simulink model "Bai6"  (R2019a)
settings: Solver=VariableStepAuto  StartTime=0.0  StopTime=10  RelTol=1e-3
libraries: commanabbnd3 x1
settings Model: Creator=ASUS  LastModifiedBy=ASUS

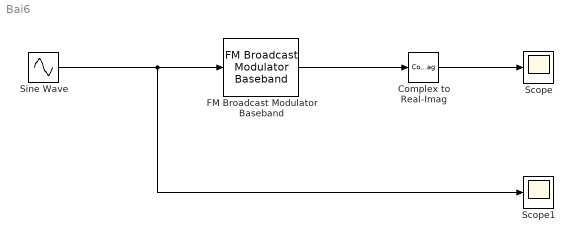
== system Bai6 ==
  Complex to Real-Imag : ComplexToRealImag  Output=Real
  FM Broadcast Modulator Baseband : commanabbnd3/FM Broadcast Modulator Baseband  SampleRate=240e3  FrequencyDeviation=100  FilterTimeConstant=75e-6  AudioSampleRate=48e3  Stereo=off  RBDS=off  RBDSSamplesPerSymbol=10  SimulateUsing=Code generation
      settings: SourceProductName=Communications Toolbox  SourceProductBaseCode=CM
  Scope : Scope
  Scope1 : Scope
  Sine Wave : Sin  Frequency=10  SampleTime=0.001
  wires:
  FM Broadcast Modulator Baseband/1 -> Complex to Real-Imag/1
  Sine Wave/1 -> Scope1/1, FM Broadcast Modulator Baseband/1
  Complex to Real-Imag/1 -> Scope/1
